simulink model "fuzzy_ruido"  (R2023a)
settings: Solver=VariableStepAuto  StartTime=0.0  StopTime=400  RelTol=1e-3
values from neighbouring files (symbols this model uses):
  A1 = 0.0154    [parametros.m]    (also in variables.mat)
  A2 = 5e-5    (= 5e-05)    [parametros.m]    (also in variables.mat)
  az = 0.5    [parametros.m]    (also in variables.mat)
  g = 9.8    [parametros.m]    (also in variables.mat)
  H_star = H_max/2    (= 0.31)    [parametros.m]    (also in variables.mat)
  Q_star = ro*A2*az*sqrt(2*g*H_star)    [parametros.m]    (also in variables.mat = 0.0616238590158)
  ro = 1000    [parametros.m]    (also in variables.mat)
undefined symbols (not defined in the file or in its folder): DiscIntNeverNeededParam
libraries: fuzblock x1
settings Model: Creator=empg0  LastModifiedBy=empg0

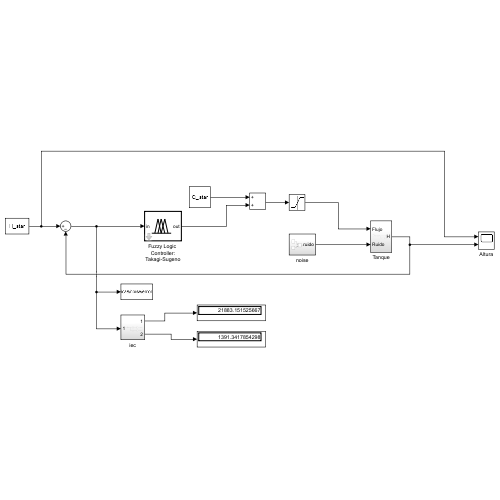
[thumbnail: Simulink's stored preview of the top-level diagram]
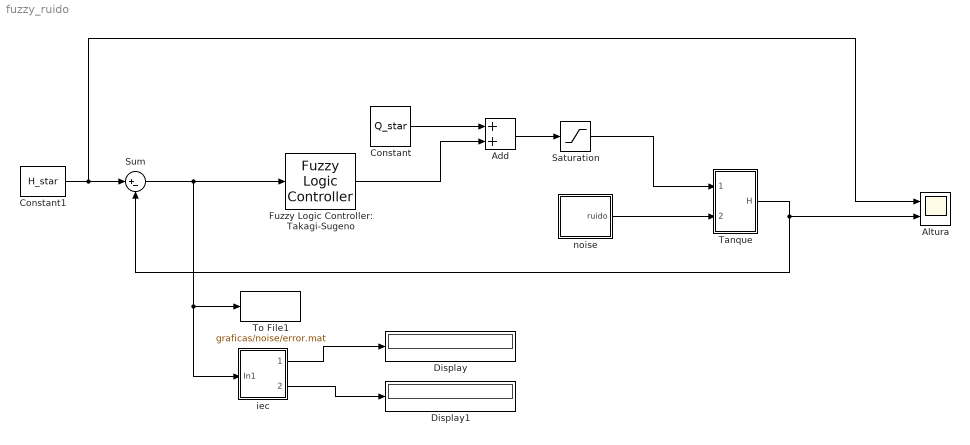
== system fuzzy_ruido ==
  Add : Sum
  Altura : Scope  NumInputPorts=2
  Constant : Constant  Value=Q_star
  Constant1 : Constant  Value=H_star
  Display : Display
  Display1 : Display
  Fuzzy Logic Controller: Takagi-Sugeno : fuzblock/Fuzzy Logic  Controller  FIS='error_fuzzy.fis'  OutputSampleNumber=101  DataType=double  FuzzifiedInputs=off  RuleFiringStrengths=off  RuleOutputs=off  AggregatedOutputs=off  SimulateUsing=Interpreted execution  OutOfRangeInputValueMessage=warning  NoRuleFiredMessage=warning  EmptyOutputFuzzySetMessage=warning
  Saturation : Saturate  UpperLimit=0.1  LowerLimit=0
  Sum : Sum  Inputs=|+-
  Tanque : Subsystem
  To File1 : ToFile  Filename=graficas/noise/error.mat  MatrixName=error  SampleTime=0.5
  iec : Subsystem
  noise : Subsystem
  wires:
  Constant/1 -> Add/1
  Tanque/1(H) -> Altura/2, Sum/2
  Sum/1 -> To File1/1, iec/1(In1), Fuzzy Logic Controller: Takagi-Sugeno/1
  Fuzzy Logic Controller: Takagi-Sugeno/1 -> Add/2
  Add/1 -> Saturation/1
  Saturation/1 -> Tanque/1(Flujo)
  Constant1/1 -> Sum/1, Altura/1
  iec/1(Out1) -> Display/1
  noise/1(ruido) -> Tanque/2(Ruido)
  iec/2(Out2) -> Display1/1

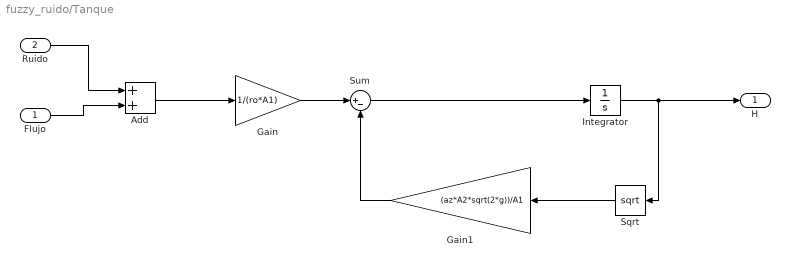
== system fuzzy_ruido/Tanque ==
  Flujo : Inport
  Ruido : Inport  Port=2
  Add : Sum
  Gain : Gain  Gain=1/(ro*A1)
  Gain1 : Gain  Gain=(az*A2*sqrt(2*g))/A1
  Integrator : Integrator  LimitOutput=on  UpperSaturationLimit=0.62  LowerSaturationLimit=0
  Sqrt : Sqrt
  Sum : Sum  Inputs=|+-
  H : Outport
  wires:
  Gain/1 -> Sum/1
  Sum/1 -> Integrator/1
  Sqrt/1 -> Gain1/1
  Gain1/1 -> Sum/2
  Integrator/1 -> H/1, Sqrt/1
  Add/1 -> Gain/1
  Flujo/1 -> Add/2
  Ruido/1 -> Add/1

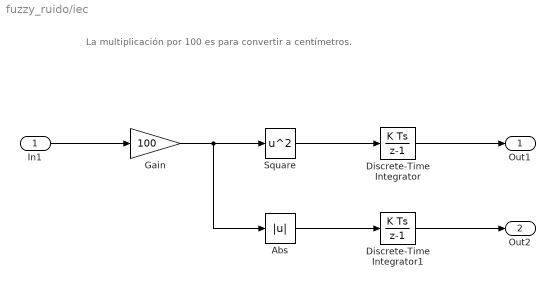
== system fuzzy_ruido/iec ==
  note: La multiplicación por 100 es para convertir a centímetros.
  In1 : Inport
  Abs : Abs  SaturateOnIntegerOverflow=off
  Discrete-Time Integrator : DiscreteIntegrator  SampleTime=0.001  ICPrevOutput=DiscIntNeverNeededParam  ICPrevScaledInput=DiscIntNeverNeededParam
  Discrete-Time Integrator1 : DiscreteIntegrator  SampleTime=0.001  ICPrevOutput=DiscIntNeverNeededParam  ICPrevScaledInput=DiscIntNeverNeededParam
  Gain : Gain  Gain=100
  Square : Math  Operator=square  SignedPower=on  RndMeth=Zero
  Out1 : Outport
  Out2 : Outport  Port=2
  wires:
  In1/1 -> Gain/1
  Gain/1 -> Abs/1, Square/1
  Square/1 -> Discrete-Time Integrator/1
  Discrete-Time Integrator/1 -> Out1/1
  Abs/1 -> Discrete-Time Integrator1/1
  Discrete-Time Integrator1/1 -> Out2/1

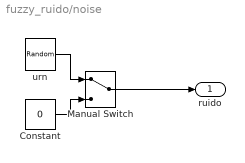
== system fuzzy_ruido/noise ==
  Constant : Constant  Value=0
  Manual Switch : ManualSwitch
  urn : UniformRandomNumber  Minimum=-0.1*0.1  Maximum=0.1*0.1  Seed=140  SampleTime=20
  ruido : Outport
  wires:
  urn/1 -> Manual Switch/1
  Constant/1 -> Manual Switch/2
  Manual Switch/1 -> ruido/1
